simulink model "SF107A_MotRplCoggCmd"  (R2013b)
settings: Solver=FixedStepDiscrete  SolverMode=SingleTasking  StartTime=0.0  StopTime=1  FixedStep=0.002  RelTol=1e-3
values from neighbouring files (symbols this model uses):
  ARCHGLBPRM_2PI_ULS_F32 = DataDict.Constant    [SF107A_MotRplCoggCmd_DataDict.m]
  ARCHGLBPRM_FLOATZEROTHD_ULS_F32 = DataDict.Constant    [SF107A_MotRplCoggCmd_DataDict.m]
  ININITRNIDXCON_CNT_U16 = DataDict.Constant    [SF107A_MotRplCoggCmd_DataDict.m]
  ITRNIDXCON_CNT_U08 = DataDict.Constant    [SF107A_MotRplCoggCmd_DataDict.m]
  MotRplCoggCmdHrmncOrder1Elec = DataDict.Calibration    [SF107A_MotRplCoggCmd_DataDict.m]
  MotRplCoggCmdHrmncOrder2Elec = DataDict.Calibration    [SF107A_MotRplCoggCmd_DataDict.m]
  MotRplCoggCmdHrmncOrder3Elec = DataDict.Calibration    [SF107A_MotRplCoggCmd_DataDict.m]
  ONEOVER12_MOTREV_F32 = DataDict.Constant    [SF107A_MotRplCoggCmd_DataDict.m]
  ONEOVER2_ULS_F32 = DataDict.Constant    [SF107A_MotRplCoggCmd_DataDict.m]
  ONEOVER2PI_ULS_F32 = DataDict.Constant    [SF107A_MotRplCoggCmd_DataDict.m]
  ONEOVER4_ULS_F32 = DataDict.Constant    [SF107A_MotRplCoggCmd_DataDict.m]
  SINCNVNCON1_ULS_F32 = DataDict.Constant    [SF107A_MotRplCoggCmd_DataDict.m]
  SINCNVNCON2_ULS_F32 = DataDict.Constant    [SF107A_MotRplCoggCmd_DataDict.m]
  SINCNVNCONTBL_ULS_U16 = DataDict.Constant    [SF107A_MotRplCoggCmd_DataDict.m]
undefined symbols (not defined in the file or in its folder): NvmGetErrSts1
libraries: FloatToFixd x8, FixdToFloat x8, NxtrNvM x3, NxtrLim x3, simulink x2, NxtrAbslt x1
(part 1 of 3)
settings Model: Creator=BZHF94  LastModifiedBy=BZHF94
settings SolverCC: AutoInsertRateTranBlk=on  InsertRTBMode=Always
settings DataIOCC: LimitDataPoints=off  SaveFormat=Structure  ReturnWorkspaceOutputs=on
settings OptimizationCC: BlockReduction=off  InlineParams=on  ZeroExternalMemoryAtStartup=off  ZeroInternalMemoryAtStartup=off  OptimizeModelRefInitCode=on  LifeSpan=1
settings DebuggingCC: SignalInfNanChecking=error  SignalRangeChecking=warning  UnderspecifiedInitializationDetection=Simplified  SolverPrmCheckMsg=error  InheritedTsInSrcMsg=error  DiscreteInheritContinuousMsg=error  SingleTaskRateTransMsg=error  TasksWithSamePriorityMsg=error  SigSpecEnsureSampleTimeMsg=error  CheckMatrixSingularityMsg=error  ParameterUnderflowMsg=error  ParameterPrecisionLossMsg=error  ParameterTunabilityLossMsg=error  FixptConstUnderflowMsg=warning  FixptConstOverflowMsg=warning  VectorMatrixConversionMsg=error  SignalLabelMismatchMsg=error  UnconnectedInputMsg=error  UnconnectedOutputMsg=error  UnconnectedLineMsg=error  SFcnCompatibilityMsg=error  UniqueDataStoreMsg=warning  BusObjectLabelMismatch=error  RootOutportRequireBusObject=error  AssertControl=DisableAll  ModelReferenceIOMsg=error  ModelReferenceVersionMismatchMessage=warning  ModelReferenceIOMismatchMessage=error  ModelReferenceCSMismatchMessage=warning  ModelReferenceDataLoggingMessage=error  StateNameClashWarn=warning  StrictBusMsg=ErrorOnBusTreatedAsVector  NonBusSignalsTreatedAsBus=error  SFUnexpectedBacktrackingDiag=error  SFInvalidInputDataAccessInChartInitDiag=error  SFNoUnconditionalDefaultTransitionDiag=error  SFTransitionOutsideNaturalParentDiag=error  SFUnconditionalTransitionShadowingDiag=error  SFUndirectedBroadcastEventsDiag=error
settings ModelReferenceCC: ModelReferenceNumInstancesAllowed=Single
settings RTWCC: SystemTargetFile=autosar.tlc  GenCodeOnly=on  TemplateMakefile=ert_default_tmf  Description=AUTOSAR  GenerateReport=on  ProcessScript=autosar_make_rtw_hook  LaunchReport=on
settings CodeAppCC: GenerateComments=off  IgnoreCustomStorageClasses=off  CustomSymbolStrType=$N$R$M  CustomSymbolStrBlkIO=$N$M  SimulinkBlockComments=off
settings STFCustomTargetCC: ParMdlRefBuildCompliant=on  CompOptLevelCompliant=on  IncludeMdlTerminateFcn=off  CombineOutputUpdateFcns=on  SuppressErrorStatus=on  ERTFirstTimeCompliant=on  ERTCustomFileBanners=on  SupportNonFinite=off  SupportComplex=off  SupportContinuousTime=off  SupportNonInlinedSFcns=off  MATLABClassNameForMDSCustomization=Simulink.SoftwareTarget.ERTCustomization  AutosarCompliant=on  GRTInterface=off  SystemTargetFile=autosar.tlc
settings ERTTargetCC: CodeReplacementLibrary=ANSI_C  ConcurrentExecutionCompliant=off  IncludeMdlTerminateFcn=off  SuppressErrorStatus=on  SupportNonFinite=off  SupportComplex=off  ModelStepFunctionPrototypeControlCompliant=off  CPPClassGenCompliant=off  AutosarCompliant=on  InlinedParameterPlacement=NonHierarchical  ERTCustomFileTemplate=example_file_process.tlc  EnableUserReplacementTypes=on

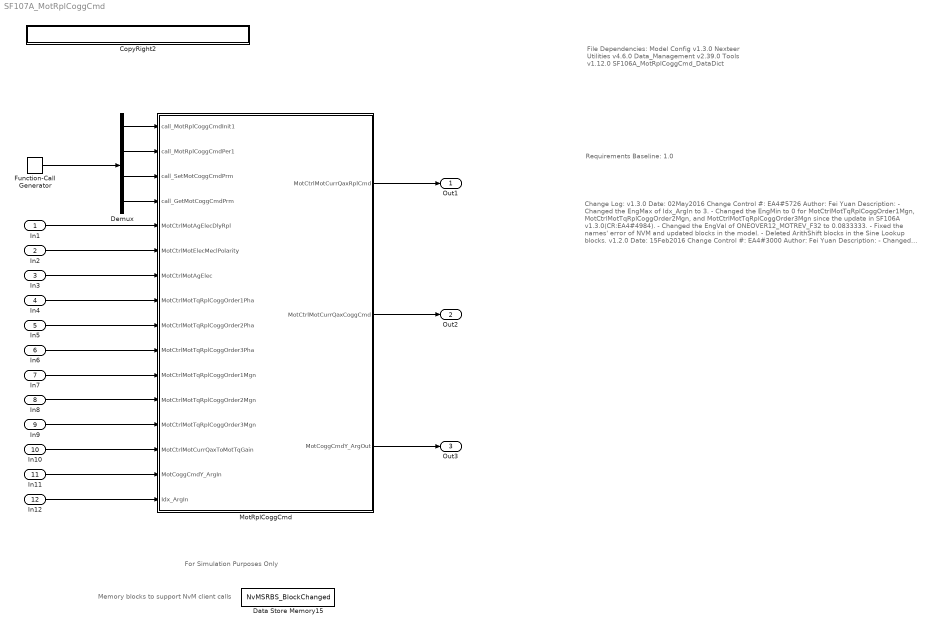
== system SF107A_MotRplCoggCmd ==
  note: Change Log:
      |
      | v1.3.0
      | Date: 02May2016
      | Change Control #: EA4#5726
      | Author: Fei Yuan
      | Description:
      | - Changed the EngMax of Idx_ArgIn to 3.
      | - Changed the EngMin to 0 for MotCtrlMotTqRplCoggOrder1Mgn,
      |   MotCtrlMotTqRplCoggOrder2Mgn, and MotCtrlMotTqRplCoggOrder3Mgn
      |   since the update in SF106A v1.3.0(CR:EA4#4984).
      | - Changed the EngVal of ONEOVER12_MOTREV_F32 to 0.0833333.
      | - Fixed the names' error of NVM and updated blocks in the model.
      | - Deleted ArithShift blocks in the Sine Lookup blocks.
      |
      |
      | v1.2.0
      | Date: 15Feb2016
      | Change Control #: EA4#3000
      | Author: Fei Yuan
      | Description:
      | - Changed the logic of wrapping block to fix the floating point exception.
      |
      |
      | v1.1.0
      | Date: 11February2016
      | Change Control #: EA4#3000
      | Author: Fei Yuan
      | Description:
      | - Change Per1 context to "Non-Rte".
      | - Add "MotRplCoggCmdInit1" to SetRamBlockStatus CallLocation
      | - Correct the MOTRPLCMDHILIM_AMPR_F32.EngMax to 29.
      | - Delete COGGIDXCON_CNT_U16 and MOTCOGGCMDY_MOTNWTMTR_S1P14
      | - Add the Constant ININITRNIDXCON_CNT_U16.
      | - Change the size of SINCNVNCONTBL_ULS_U16 to 513.
      | - Add a missed unary block.
      | - Add new logic in "Convert to 0 to Pi/2" block.
      |
      |
      | v1.0.0
      | Date: 01February2016
      | Change Control #: EA4#3000
      | Author: Fei Yuan
      | Description:
      | - Initial release for EA4 based on version 1 in EA3.
  note: File Dependencies:
      |
      | Model Config v1.3.0
      | Nexteer Utilities v4.6.0
      | Data_Management v2.39.0
      | Tools v1.12.0
      | SF106A_MotRplCoggCmd_DataDict
  note: Requirements Baseline: 1.0
  note: For Simulation Purposes Only
  note: Memory blocks to support NvM client calls
  In1 : Inport
  In2 : Inport  Port=2
  In3 : Inport  Port=3
  In4 : Inport  Port=4
  In5 : Inport  Port=5
  In6 : Inport  Port=6
  In7 : Inport  Port=7
  In8 : Inport  Port=8
  In9 : Inport  Port=9
  In10 : Inport  Port=10
  In11 : Inport  Port=11  OutDataTypeStr=int16
  In12 : Inport  Port=12
  CopyRight2 : Subsystem  Description=|  mask(Copyright Information){none=on}
      | Copyright info block.                                               
      |                                                                     
      | Place copyright information at the top of every subsystem in design.
      mask prompts: none "No parameters"
      mask help: Place copyright information at the top of every subsystem in design.
      mask Display:
      | NxtrConf = 'Nexteer Confidential';
      | 
      | sys = bdroot; %handle for the current model ("system")
      | first = get_param(sys,'Created');
      | if(isempty(first))
      |     first = datestr(now,'yyyy');
      | else
      |     first = first(end-3:end);  %year is last four digits
      | end
      | 
      | last = get_param(sys,'LastModifiedDate');
      | if isempty(last)
      |     last = datestr(now,'yyyy');
      | else
      |     last = last(end-3:end);
      | end
      | 
      | if strcmp(first,last)
      |     fprintf('%s -- Copyright %s Nexteer',NxtrConf,first)
      | else
      |     fprintf('%s -- %s%s- %s Nexteer',NxtrConf,char(169),first,last)
      | end
  Data Store Memory15 : DataStoreMemory  DataStoreName=NvMSRBS_BlockChanged  VectorParams1D=off
  Demux : Demux
  Function-Call Generator : simulink/Ports & Subsystems/Function-Call Generator  RequirementInfo={} %GIDa_6477a55e_09d1_416c_bd2a_f96e072289e0  sample_time=1  numberOfIterations=1
  MotRplCoggCmd : Subsystem
  Out1 : Outport
  Out2 : Outport  Port=2
  Out3 : Outport  Port=3
  wires:
  In1/1 -> MotRplCoggCmd/5(MotCtrlMotAgElecDlyRpl)
  In2/1 -> MotRplCoggCmd/6(MotCtrlMotElecMeclPolarity)
  In3/1 -> MotRplCoggCmd/7(MotCtrlMotAgElec)
  In4/1 -> MotRplCoggCmd/8(MotCtrlMotTqRplCoggOrder1Pha)
  In5/1 -> MotRplCoggCmd/9(MotCtrlMotTqRplCoggOrder2Pha)
  In6/1 -> MotRplCoggCmd/10(MotCtrlMotTqRplCoggOrder3Pha)
  In7/1 -> MotRplCoggCmd/11(MotCtrlMotTqRplCoggOrder1Mgn)
  In8/1 -> MotRplCoggCmd/12(MotCtrlMotTqRplCoggOrder2Mgn)
  In9/1 -> MotRplCoggCmd/13(MotCtrlMotTqRplCoggOrder3Mgn)
  In10/1 -> MotRplCoggCmd/14(MotCtrlMotCurrQaxToMotTqGain)
  MotRplCoggCmd/1(MotCtrlMotCurrQaxRplCmd) -> Out1/1
  MotRplCoggCmd/2(MotCtrlMotCurrQaxCoggCmd) -> Out2/1
  Function-Call Generator/1 -> Demux/1
  In11/1 -> MotRplCoggCmd/15(MotCoggCmdY_ArgIn)
  In12/1 -> MotRplCoggCmd/16(Idx_ArgIn)
  Demux/3 -> MotRplCoggCmd/3(call_SetMotCoggCmdPrm)
  Demux/4 -> MotRplCoggCmd/4(call_GetMotCoggCmdPrm)
  Demux/2 -> MotRplCoggCmd/2(call_MotRplCoggCmdPer1)
  Demux/1 -> MotRplCoggCmd/1(call_MotRplCoggCmdInit1)
  MotRplCoggCmd/3(MotCoggCmdY_ArgOut) -> Out3/1

== system SF107A_MotRplCoggCmd/CopyRight2 ==

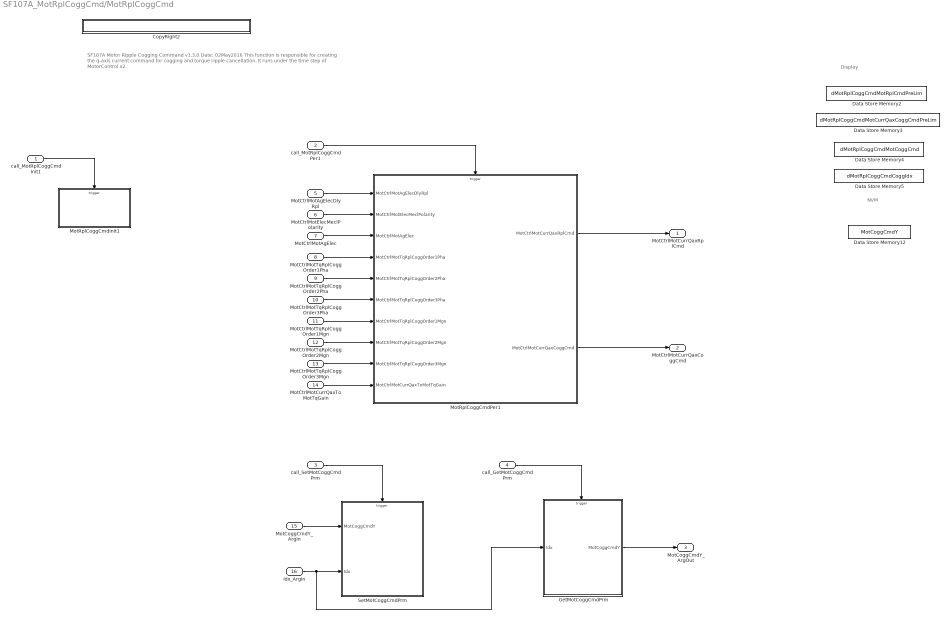
== system SF107A_MotRplCoggCmd/MotRplCoggCmd ==
  note: SF107A  Motor Ripple Cogging Command
      | v1.3.0      Date: 02May2016
      |
      | This function is responsible for creating the q-axis current command for cogging and torque ripple cancellation.
      | It runs under the time step of MotorControl x2.
  note: NVM
  note: Display
  call_MotRplCoggCmdInit1 : Inport
  call_MotRplCoggCmdPer1 : Inport  RequirementInfo="{'linktype_rmi_doors' '0000bb46 (/E-STEER Core/SubSystem Specifications/Application Functions/SF99/SF107A Cogging and Ripple Command Generation)' '#SF107A_49' 'true' 'REQ:  SF107A_49' '' } %GIDa_bcde757e_fcf1_400f_9a5c_d951bd685b53"  Port=2
  call_SetMotCoggCmdPrm : Inport  Port=3
  call_GetMotCoggCmdPrm : Inport  Port=4
  MotCtrlMotAgElecDlyRpl : Inport  RequirementInfo="{'linktype_rmi_doors' '0000bb46 (/E-STEER Core/SubSystem Specifications/Application Functions/SF99/SF107A Cogging and Ripple Command Generation)' '#SF107A_45' 'true' 'REQ:  SF107A_45' '' } %GIDa_759bd4cf_ee1e_4f48_ad2a_68232b25c211"  Port=5
  MotCtrlMotElecMeclPolarity : Inport  RequirementInfo="{'linktype_rmi_doors' '0000bb46 (/E-STEER Core/SubSystem Specifications/Application Functions/SF99/SF107A Cogging and Ripple Command Generation)' '#SF107A_46' 'true' 'REQ:  SF107A_46' '' } %GIDa_d359bdf1_f0a3_4952_a26e_4e6f5812eb7c"  Port=6
  MotCtrlMotAgElec : Inport  RequirementInfo="{'linktype_rmi_doors' '0000bb46 (/E-STEER Core/SubSystem Specifications/Application Functions/SF99/SF107A Cogging and Ripple Command Generation)' '#SF107A_43' 'true' 'REQ:  SF107A_43' '' } %GIDa_21806179_a7db_45e0_974d_baa248ff84af"  Port=7
  MotCtrlMotTqRplCoggOrder1Pha : Inport  RequirementInfo="{'linktype_rmi_doors' '0000bb46 (/E-STEER Core/SubSystem Specifications/Application Functions/SF99/SF107A Cogging and Ripple Command Generation)' '#SF107A_38' 'true' 'REQ:  SF107A_38' '' } %GIDa_76ec82d2_a38c_47ae_b701_241d2d548300"  Port=8
  MotCtrlMotTqRplCoggOrder2Pha : Inport  RequirementInfo="{'linktype_rmi_doors' '0000bb46 (/E-STEER Core/SubSystem Specifications/Application Functions/SF99/SF107A Cogging and Ripple Command Generation)' '#SF107A_40' 'true' 'REQ:  SF107A_40' '' } %GIDa_59edcd68_ad99_42db_8c02_5e556eb509ac"  Port=9
  MotCtrlMotTqRplCoggOrder3Pha : Inport  RequirementInfo="{'linktype_rmi_doors' '0000bb46 (/E-STEER Core/SubSystem Specifications/Application Functions/SF99/SF107A Cogging and Ripple Command Generation)' '#SF107A_42' 'true' 'REQ:  SF107A_42' '' } %GIDa_4883dac2_53a7_4d05_a76a_d63a8a01ae4d"  Port=10
  MotCtrlMotTqRplCoggOrder1Mgn : Inport  RequirementInfo="{'linktype_rmi_doors' '0000bb46 (/E-STEER Core/SubSystem Specifications/Application Functions/SF99/SF107A Cogging and Ripple Command Generation)' '#SF107A_27' 'true' 'REQ:  SF107A_27' '' } %GIDa_75ad0a99_38bc_44be_af39_747cf86f05ec"  Port=11
  MotCtrlMotTqRplCoggOrder2Mgn : Inport  RequirementInfo="{'linktype_rmi_doors' '0000bb46 (/E-STEER Core/SubSystem Specifications/Application Functions/SF99/SF107A Cogging and Ripple Command Generation)' '#SF107A_39' 'true' 'REQ:  SF107A_39' '' } %GIDa_040945aa_cac7_4d8d_86dc_7274d12a7576"  Port=12
  MotCtrlMotTqRplCoggOrder3Mgn : Inport  RequirementInfo="{'linktype_rmi_doors' '0000bb46 (/E-STEER Core/SubSystem Specifications/Application Functions/SF99/SF107A Cogging and Ripple Command Generation)' '#SF107A_41' 'true' 'REQ:  SF107A_41' '' } %GIDa_1dbb5808_0eab_4535_8b60_cc6f49189c56"  Port=13
  MotCtrlMotCurrQaxToMotTqGain : Inport  RequirementInfo="{'linktype_rmi_doors' '0000bb46 (/E-STEER Core/SubSystem Specifications/Application Functions/SF99/SF107A Cogging and Ripple Command Generation)' '#SF107A_44' 'true' 'REQ:  SF107A_44' '' } %GIDa_8093fd36_868b_4102_b9e2_e2b5f3d0e07d"  Port=14
  MotCoggCmdY_ArgIn : Inport  Port=15
  Idx_ArgIn : Inport  Port=16
  CopyRight2 : Subsystem  Description=|  mask(Copyright Information){none=on}
      | Copyright info block.                                               
      |                                                                     
      | Place copyright information at the top of every subsystem in design.
      mask prompts: none "No parameters"
      mask help: Place copyright information at the top of every subsystem in design.
      mask Display:
      | NxtrConf = 'Nexteer Confidential';
      | 
      | sys = bdroot; %handle for the current model ("system")
      | first = get_param(sys,'Created');
      | if(isempty(first))
      |     first = datestr(now,'yyyy');
      | else
      |     first = first(end-3:end);  %year is last four digits
      | end
      | 
      | last = get_param(sys,'LastModifiedDate');
      | if isempty(last)
      |     last = datestr(now,'yyyy');
      | else
      |     last = last(end-3:end);
      | end
      | 
      | if strcmp(first,last)
      |     fprintf('%s -- Copyright %s Nexteer',NxtrConf,first)
      | else
      |     fprintf('%s -- %s%s- %s Nexteer',NxtrConf,char(169),first,last)
      | end
  Data Store Memory12 : DataStoreMemory  DataStoreName=MotCoggCmdY  InitialValue=[]  OutDataTypeStr=int16  StateMustResolveToSignalObject=on
  Data Store Memory2 : DataStoreMemory  DataStoreName=dMotRplCoggCmdMotRplCmdPreLim  InitialValue=[]  VectorParams1D=off  StateMustResolveToSignalObject=on
  Data Store Memory3 : DataStoreMemory  DataStoreName=dMotRplCoggCmdMotCurrQaxCoggCmdPreLim  InitialValue=[]  VectorParams1D=off  StateMustResolveToSignalObject=on
  Data Store Memory4 : DataStoreMemory  DataStoreName=dMotRplCoggCmdMotCoggCmd  InitialValue=[]  VectorParams1D=off  StateMustResolveToSignalObject=on
  Data Store Memory5 : DataStoreMemory  DataStoreName=dMotRplCoggCmdCoggIdx  InitialValue=[]  VectorParams1D=off  StateMustResolveToSignalObject=on
  GetMotCoggCmdPrm : Subsystem
  MotRplCoggCmdInit1 : Subsystem
  MotRplCoggCmdPer1 : Subsystem
  SetMotCoggCmdPrm : Subsystem
  MotCtrlMotCurrQaxRplCmd : Outport  RequirementInfo="{'linktype_rmi_doors' '0000bb46 (/E-STEER Core/SubSystem Specifications/Application Functions/SF99/SF107A Cogging and Ripple Command Generation)' '#SF107A_47' 'true' 'REQ:  SF107A_47' '' } %GIDa_c223fd26_86db_4771_9987_8f6635ad3f76"
  MotCtrlMotCurrQaxCoggCmd : Outport  RequirementInfo="{'linktype_rmi_doors' '0000bb46 (/E-STEER Core/SubSystem Specifications/Application Functions/SF99/SF107A Cogging and Ripple Command Generation)' '#SF107A_28' 'true' 'REQ:  SF107A_28' '' } %GIDa_efe72f72_a005_42fa_9193_c14ee39dea59"  Port=2
  MotCoggCmdY_ArgOut : Outport  Port=3
  wires:
  MotCtrlMotAgElecDlyRpl/1 -> MotRplCoggCmdPer1/1(MotCtrlMotAgElecDlyRpl)
  MotCtrlMotElecMeclPolarity/1 -> MotRplCoggCmdPer1/2(MotCtrlMotElecMeclPolarity)
  MotCtrlMotAgElec/1 -> MotRplCoggCmdPer1/3(MotCtrlMotAgElec)
  MotCtrlMotTqRplCoggOrder1Pha/1 -> MotRplCoggCmdPer1/4(MotCtrlMotTqRplCoggOrder1Pha)
  MotCtrlMotTqRplCoggOrder2Pha/1 -> MotRplCoggCmdPer1/5(MotCtrlMotTqRplCoggOrder2Pha)
  MotCtrlMotTqRplCoggOrder3Pha/1 -> MotRplCoggCmdPer1/6(MotCtrlMotTqRplCoggOrder3Pha)
  MotCtrlMotTqRplCoggOrder1Mgn/1 -> MotRplCoggCmdPer1/7(MotCtrlMotTqRplCoggOrder1Mgn)
  MotCtrlMotTqRplCoggOrder2Mgn/1 -> MotRplCoggCmdPer1/8(MotCtrlMotTqRplCoggOrder2Mgn)
  MotCtrlMotTqRplCoggOrder3Mgn/1 -> MotRplCoggCmdPer1/9(MotCtrlMotTqRplCoggOrder3Mgn)
  MotCtrlMotCurrQaxToMotTqGain/1 -> MotRplCoggCmdPer1/10(MotCtrlMotCurrQaxToMotTqGain)
  MotRplCoggCmdPer1/1(MotCtrlMotCurrQaxRplCmd) -> MotCtrlMotCurrQaxRplCmd/1
  MotRplCoggCmdPer1/2(MotCtrlMotCurrQaxCoggCmd) -> MotCtrlMotCurrQaxCoggCmd/1
  call_MotRplCoggCmdPer1/1 -> MotRplCoggCmdPer1/Trigger
  call_MotRplCoggCmdInit1/1 -> MotRplCoggCmdInit1/Trigger
  call_SetMotCoggCmdPrm/1 -> SetMotCoggCmdPrm/Trigger
  call_GetMotCoggCmdPrm/1 -> GetMotCoggCmdPrm/Trigger
  Idx_ArgIn/1 -> GetMotCoggCmdPrm/1(Idx), SetMotCoggCmdPrm/2(Idx)
  MotCoggCmdY_ArgIn/1 -> SetMotCoggCmdPrm/1(MotCoggCmdY)
  GetMotCoggCmdPrm/1(MotCoggCmdY) -> MotCoggCmdY_ArgOut/1

== system SF107A_MotRplCoggCmd/MotRplCoggCmd/CopyRight2 ==

== system SF107A_MotRplCoggCmd/MotRplCoggCmd/GetMotCoggCmdPrm ==
  Idx : Inport
  function : TriggerPort  TriggerType=function-call
  Constant1 : Constant  Value=ITRNIDXCON_CNT_U08  OutDataTypeStr=int16
  CopyRight1 : Subsystem  Description=|  mask(Copyright Information){none=on}
      | Copyright info block.                                               
      |                                                                     
      | Place copyright information at the top of every subsystem in design.
      mask prompts: none "No parameters"
      mask help: Place copyright information at the top of every subsystem in design.
      mask Display:
      | NxtrConf = 'Nexteer Confidential';
      | 
      | sys = bdroot; %handle for the current model ("system")
      | first = get_param(sys,'Created');
      | if(isempty(first))
      |     first = datestr(now,'yyyy');
      | else
      |     first = first(end-3:end);  %year is last four digits
      | end
      | 
      | last = get_param(sys,'LastModifiedDate');
      | if isempty(last)
      |     last = datestr(now,'yyyy');
      | else
      |     last = last(end-3:end);
      | end
      | 
      | if strcmp(first,last)
      |     fprintf('%s -- Copyright %s Nexteer',NxtrConf,first)
      | else
      |     fprintf('%s -- %s%s- %s Nexteer',NxtrConf,char(169),first,last)
      | end
  For Iterator Subsystem : Subsystem  RequirementInfo="{'linktype_rmi_doors' '0000bb46 (/E-STEER Core/SubSystem Specifications/Application Functions/SF99/SF107A Cogging and Ripple Command Generation)' '#SF107A_33' 'true' 'REQ:  SF107A_33' '' } %GIDa_45473554_817e_49b7_8dca_101340bc12f0"  TreatAsAtomicUnit=on
  MotCoggCmdY : Outport
  wires:
  Idx/1 -> For Iterator Subsystem/1(Idx)
  For Iterator Subsystem/1(MotCoggCmdY) -> MotCoggCmdY/1
  Constant1/1 -> For Iterator Subsystem/2(ItrnIdxCon)

== system SF107A_MotRplCoggCmd/MotRplCoggCmd/MotRplCoggCmdInit1 ==
  function : TriggerPort  TriggerType=function-call
  CopyRight2 : Subsystem  Description=|  mask(Copyright Information){none=on}
      | Copyright info block.                                               
      |                                                                     
      | Place copyright information at the top of every subsystem in design.
      mask prompts: none "No parameters"
      mask help: Place copyright information at the top of every subsystem in design.
      mask Display:
      | NxtrConf = 'Nexteer Confidential';
      | 
      | sys = bdroot; %handle for the current model ("system")
      | first = get_param(sys,'Created');
      | if(isempty(first))
      |     first = datestr(now,'yyyy');
      | else
      |     first = first(end-3:end);  %year is last four digits
      | end
      | 
      | last = get_param(sys,'LastModifiedDate');
      | if isempty(last)
      |     last = datestr(now,'yyyy');
      | else
      |     last = last(end-3:end);
      | end
      | 
      | if strcmp(first,last)
      |     fprintf('%s -- Copyright %s Nexteer',NxtrConf,first)
      | else
      |     fprintf('%s -- %s%s- %s Nexteer',NxtrConf,char(169),first,last)
      | end
  Data Type Conversion : DataTypeConversion  RequirementInfo="{'linktype_rmi_doors' '0000bb46 (/E-STEER Core/SubSystem Specifications/Application Functions/SF99/SF107A Cogging and Ripple Command Generation)' '#SF107A_61' 'true' 'REQ:  SF107A_61' '' } %GIDa_7543bd06_1602_4119_b52d_e662400f79a4"  OutDataTypeStr=int32
  Data Type Conversion1 : DataTypeConversion  RequirementInfo="{'linktype_rmi_doors' '0000bb46 (/E-STEER Core/SubSystem Specifications/Application Functions/SF99/SF107A Cogging and Ripple Command Generation)' '#SF107A_61' 'true' 'REQ:  SF107A_61' '' } %GIDa_e4f111be_1c13_4101_a6fe_36d4dd11c4c4"  OutDataTypeStr=Enum: NvmGetErrSts1
  Enumerated Constant : simulink/Sources/Enumerated Constant  RequirementInfo="{'linktype_rmi_doors' '0000bb46 (/E-STEER Core/SubSystem Specifications/Application Functions/SF99/SF107A Cogging and Ripple Command Generation)' '#SF107A_61' 'true' 'REQ:  SF107A_61' '' } %GIDa_6ad17a04_5c1e_4dc7_8ab4_71a48d0dc388"  OutDataTypeStr=Enum: NvmGetErrSts1  Value=NvmGetErrSts1.REQUEST_OK  SampleTime=inf
  Get Error Status : NxtrNvM/Get Error Status  RequirementInfo="{'linktype_rmi_doors' '0000bb46 (/E-STEER Core/SubSystem Specifications/Application Functions/SF99/SF107A Cogging and Ripple Command Generation)' '#SF107A_61' 'true' 'REQ:  SF107A_61' '' } %GIDa_e572d21d_63bd_432d_baf2_5c021ad23777"  FuncName=Get Error Status  NvMBlockName=MotCoggCmdY  VoidFuncRtn=on  ReqResPtr_DSN=NvMGES_ReqResPtr  Return_DSN=NvMGES_ReqResPtr
      settings: AttributesFormatString=%<FuncName>
  If : If  RequirementInfo="{'linktype_rmi_doors' '0000bb46 (/E-STEER Core/SubSystem Specifications/Application Functions/SF99/SF107A Cogging and Ripple Command Generation)' '#SF107A_61' 'true' 'REQ:  SF107A_61' '' } %GIDa_e4fe0c89_1c6e_4333_af03_6094cd431682"  IfExpression=u1  ShowElse=off
  NVM is NOT okay : Subsystem  RequirementInfo="{'linktype_rmi_doors' '0000bb46 (/E-STEER Core/SubSystem Specifications/Application Functions/SF99/SF107A Cogging and Ripple Command Generation)' '#SF107A_61' 'true' 'REQ:  SF107A_61' '' } %GIDa_2b24311b_dea0_4c39_b838_f46fba703cea"  TreatAsAtomicUnit=on
  Relational Operator : RelationalOperator  RequirementInfo="{'linktype_rmi_doors' '0000bb46 (/E-STEER Core/SubSystem Specifications/Application Functions/SF99/SF107A Cogging and Ripple Command Generation)' '#SF107A_61' 'true' 'REQ:  SF107A_61' '' } %GIDa_be3389a3_2489_4935_b3c7_7ac566e8e832"  Operator=~=  OutDataTypeStr=boolean
  wires:
  Get Error Status/1 -> Data Type Conversion/1
  If/1 -> NVM is NOT okay/Action
  Enumerated Constant/1 -> Relational Operator/2
  Relational Operator/1 -> If/1
  Data Type Conversion/1 -> Data Type Conversion1/1
  Data Type Conversion1/1 -> Relational Operator/1

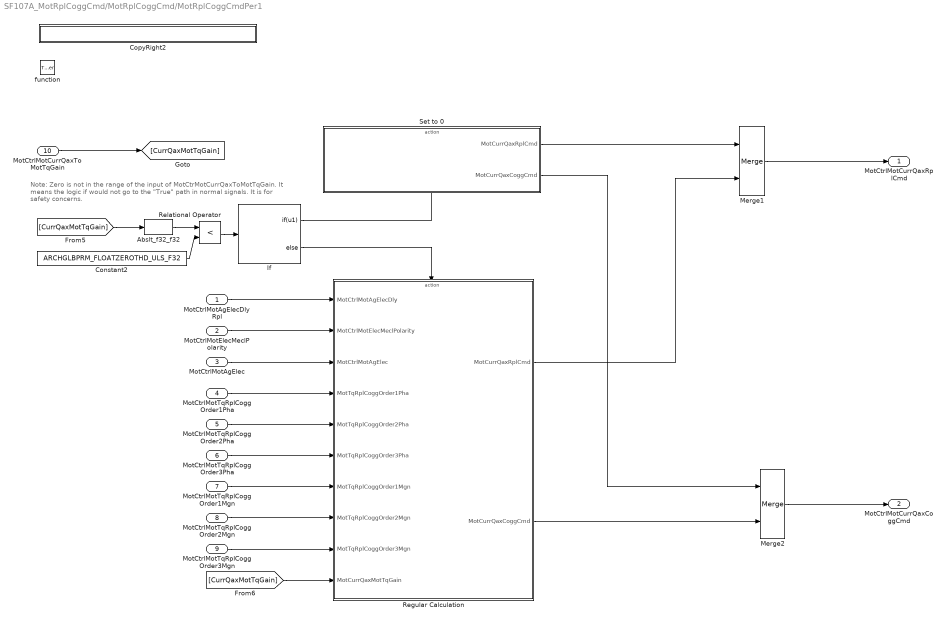
== system SF107A_MotRplCoggCmd/MotRplCoggCmd/MotRplCoggCmdPer1 ==
  note: Note: Zero is not in the range of the input of MotCtrMotCurrQaxToMotTqGain.
      | It means the logic if would not go to the "True" path in normal signals. It is for
      | safety concerns.
  MotCtrlMotAgElecDlyRpl : Inport
  MotCtrlMotElecMeclPolarity : Inport  Port=2
  MotCtrlMotAgElec : Inport  Port=3
  MotCtrlMotTqRplCoggOrder1Pha : Inport  Port=4
  MotCtrlMotTqRplCoggOrder2Pha : Inport  Port=5
  MotCtrlMotTqRplCoggOrder3Pha : Inport  Port=6
  MotCtrlMotTqRplCoggOrder1Mgn : Inport  Port=7
  MotCtrlMotTqRplCoggOrder2Mgn : Inport  Port=8
  MotCtrlMotTqRplCoggOrder3Mgn : Inport  Port=9
  MotCtrlMotCurrQaxToMotTqGain : Inport  Port=10
  function : TriggerPort  TriggerType=function-call
  Abslt_f32_f32 : NxtrAbslt/Abslt_f32_f32  RequirementInfo="{'linktype_rmi_doors' '0000bb46 (/E-STEER Core/SubSystem Specifications/Application Functions/SF99/SF107A Cogging and Ripple Command Generation)' '#SF107A_61' 'true' 'REQ:  SF107A_61' '' } %GIDa_98ab6231_9957_4905_8685_e5740981592e"  SFunctionSpec=single y1 = Abslt_f32_f32(single u1)
      settings: AttributesFormatString=%<Name>
  Constant2 : Constant  RequirementInfo="{'linktype_rmi_doors' '0000bb46 (/E-STEER Core/SubSystem Specifications/Application Functions/SF99/SF107A Cogging and Ripple Command Generation)' '#SF107A_61' 'true' 'REQ:  SF107A_61' '' } %GIDa_2b46aefd_770c_4243_8404_9e28f4c01df7"  Value=ARCHGLBPRM_FLOATZEROTHD_ULS_F32
  CopyRight2 : Subsystem  Description=|  mask(Copyright Information){none=on}
      | Copyright info block.                                               
      |                                                                     
      | Place copyright information at the top of every subsystem in design.
      mask prompts: none "No parameters"
      mask help: Place copyright information at the top of every subsystem in design.
      mask Display:
      | NxtrConf = 'Nexteer Confidential';
      | 
      | sys = bdroot; %handle for the current model ("system")
      | first = get_param(sys,'Created');
      | if(isempty(first))
      |     first = datestr(now,'yyyy');
      | else
      |     first = first(end-3:end);  %year is last four digits
      | end
      | 
      | last = get_param(sys,'LastModifiedDate');
      | if isempty(last)
      |     last = datestr(now,'yyyy');
      | else
      |     last = last(end-3:end);
      | end
      | 
      | if strcmp(first,last)
      |     fprintf('%s -- Copyright %s Nexteer',NxtrConf,first)
      | else
      |     fprintf('%s -- %s%s- %s Nexteer',NxtrConf,char(169),first,last)
      | end
  If : If  RequirementInfo="{'linktype_rmi_doors' '0000bb46 (/E-STEER Core/SubSystem Specifications/Application Functions/SF99/SF107A Cogging and Ripple Command Generation)' '#SF107A_61' 'true' 'REQ:  SF107A_61' '' } %GIDa_3a5860a3_0e2e_4331_aab2_e5b66dff5352"  IfExpression=u1
  Merge1 : Merge  RequirementInfo="{'linktype_rmi_doors' '0000bb46 (/E-STEER Core/SubSystem Specifications/Application Functions/SF99/SF107A Cogging and Ripple Command Generation)' '#SF107A_61' 'true' 'REQ:  SF107A_61' '' } %GIDa_c1020c94_da0e_48f1_812f_751dd1c0e521"
  Merge2 : Merge  RequirementInfo="{'linktype_rmi_doors' '0000bb46 (/E-STEER Core/SubSystem Specifications/Application Functions/SF99/SF107A Cogging and Ripple Command Generation)' '#SF107A_61' 'true' 'REQ:  SF107A_61' '' } %GIDa_d62df4b8_5fb9_4378_80e2_de7400452455"
  Regular Calculation : Subsystem  TreatAsAtomicUnit=on
  Relational Operator : RelationalOperator  RequirementInfo="{'linktype_rmi_doors' '0000bb46 (/E-STEER Core/SubSystem Specifications/Application Functions/SF99/SF107A Cogging and Ripple Command Generation)' '#SF107A_61' 'true' 'REQ:  SF107A_61' '' } %GIDa_0649a214_7cff_4b5d_92b0_ac2271458f93"  Operator=<  OutDataTypeStr=boolean
  Set to 0 : Subsystem  RequirementInfo="{'linktype_rmi_doors' '0000bb46 (/E-STEER Core/SubSystem Specifications/Application Functions/SF99/SF107A Cogging and Ripple Command Generation)' '#SF107A_61' 'true' 'REQ:  SF107A_61' '' } %GIDa_9ff30e71_4fe0_4a1e_8972_6be45b96b5b5"  TreatAsAtomicUnit=on
  MotCtrlMotCurrQaxRplCmd : Outport
  MotCtrlMotCurrQaxCoggCmd : Outport  Port=2
  wires:
  [CurrQaxMotTqGain] -> Abslt_f32_f32/1
  If/1 -> Set to 0/Action
  If/2 -> Regular Calculation/Action
  Merge1/1 -> MotCtrlMotCurrQaxRplCmd/1
  Merge2/1 -> MotCtrlMotCurrQaxCoggCmd/1
  MotCtrlMotAgElecDlyRpl/1 -> Regular Calculation/1(MotCtrlMotAgElecDly)
  MotCtrlMotElecMeclPolarity/1 -> Regular Calculation/2(MotCtrlMotElecMeclPolarity)
  MotCtrlMotAgElec/1 -> Regular Calculation/3(MotCtrlMotAgElec)
  [CurrQaxMotTqGain] -> Regular Calculation/10(MotCurrQaxMotTqGain)
  MotCtrlMotTqRplCoggOrder1Pha/1 -> Regular Calculation/4(MotTqRplCoggOrder1Pha)
  MotCtrlMotTqRplCoggOrder2Pha/1 -> Regular Calculation/5(MotTqRplCoggOrder2Pha)
  MotCtrlMotTqRplCoggOrder2Mgn/1 -> Regular Calculation/8(MotTqRplCoggOrder2Mgn)
  MotCtrlMotTqRplCoggOrder3Mgn/1 -> Regular Calculation/9(MotTqRplCoggOrder3Mgn)
  MotCtrlMotTqRplCoggOrder1Mgn/1 -> Regular Calculation/7(MotTqRplCoggOrder1Mgn)
  MotCtrlMotTqRplCoggOrder3Pha/1 -> Regular Calculation/6(MotTqRplCoggOrder3Pha)
  Set to 0/1(MotCurrQaxRplCmd) -> Merge1/1
  Set to 0/2(MotCurrQaxCoggCmd) -> Merge2/1
  Regular Calculation/1(MotCurrQaxRplCmd) -> Merge1/2
  Regular Calculation/2(MotCurrQaxCoggCmd) -> Merge2/2
  MotCtrlMotCurrQaxToMotTqGain/1 -> [CurrQaxMotTqGain]
  Constant2/1 -> Relational Operator/2
  Relational Operator/1 -> If/1
  Abslt_f32_f32/1 -> Relational Operator/1

== system SF107A_MotRplCoggCmd/MotRplCoggCmd/SetMotCoggCmdPrm ==
  MotCoggCmdY : Inport
  Idx : Inport  Port=2
  function : TriggerPort  TriggerType=function-call
  Constant : Constant  RequirementInfo="{'linktype_rmi_doors' '0000bb46 (/E-STEER Core/SubSystem Specifications/Application Functions/SF99/SF107A Cogging and Ripple Command Generation)' '#SF107A_61' 'true' 'REQ:  SF107A_61' '' } %GIDa_b2ba887a_b6a1_4ade_ae65_3d5e35303afc"  OutDataTypeStr=double
      settings: AttributesFormatString=%<OutDataTypeStr>
  Constant1 : Constant  Value=ITRNIDXCON_CNT_U08  OutDataTypeStr=int16
  CopyRight1 : Subsystem  Description=|  mask(Copyright Information){none=on}
      | Copyright info block.                                               
      |                                                                     
      | Place copyright information at the top of every subsystem in design.
      mask prompts: none "No parameters"
      mask help: Place copyright information at the top of every subsystem in design.
      mask Display:
      | NxtrConf = 'Nexteer Confidential';
      | 
      | sys = bdroot; %handle for the current model ("system")
      | first = get_param(sys,'Created');
      | if(isempty(first))
      |     first = datestr(now,'yyyy');
      | else
      |     first = first(end-3:end);  %year is last four digits
      | end
      | 
      | last = get_param(sys,'LastModifiedDate');
      | if isempty(last)
      |     last = datestr(now,'yyyy');
      | else
      |     last = last(end-3:end);
      | end
      | 
      | if strcmp(first,last)
      |     fprintf('%s -- Copyright %s Nexteer',NxtrConf,first)
      | else
      |     fprintf('%s -- %s%s- %s Nexteer',NxtrConf,char(169),first,last)
      | end
  For Iterator Subsystem1 : Subsystem  RequirementInfo="{'linktype_rmi_doors' '0000bb46 (/E-STEER Core/SubSystem Specifications/Application Functions/SF99/SF107A Cogging and Ripple Command Generation)' '#SF107A_32' 'true' 'REQ:  SF107A_32' '' } %GIDa_428cf9f1_ea1c_4fc8_a84e_dba4a10a7f1f"  TreatAsAtomicUnit=on
  Set Ram Block Status : NxtrNvM/Set Ram Block Status  RequirementInfo="{'linktype_rmi_doors' '0000bb46 (/E-STEER Core/SubSystem Specifications/Application Functions/SF99/SF107A Cogging and Ripple Command Generation)' '#SF107A_61' 'true' 'REQ:  SF107A_61' '' } %GIDa_b8a29836_1b5e_408e_b699_aa38fbb79f42"  FuncName=Set Ram Block Status  NvMBlockName=MotCoggCmdY  VoidFuncRtn=on  BlockChanged_DSN=NvMSRBS_BlockChanged  Return_DSN=NvMSRBS_Return
      settings: AttributesFormatString=%<FuncName>
  wires:
  Idx/1 -> For Iterator Subsystem1/2(Idx)
  Constant/1 -> Set Ram Block Status/1
  MotCoggCmdY/1 -> For Iterator Subsystem1/1(MotCoggCmdY)
  Constant1/1 -> For Iterator Subsystem1/3(ItrnIdxCon)

== system SF107A_MotRplCoggCmd/MotRplCoggCmd/GetMotCoggCmdPrm/CopyRight1 ==

== system SF107A_MotRplCoggCmd/MotRplCoggCmd/GetMotCoggCmdPrm/For Iterator Subsystem ==
  Idx : Inport
  ItrnIdxCon : Inport  Port=2
  Add : Sum
  Assignment : Assignment  IndexMode=Zero-based  OutputInitialize=Specify size for each dimension in table  IndexOptions=Index vector (port)  Indices=1  OutputSizes=128
  CopyRight1 : Subsystem  Description=|  mask(Copyright Information){none=on}
      | Copyright info block.                                               
      |                                                                     
      | Place copyright information at the top of every subsystem in design.
      mask prompts: none "No parameters"
      mask help: Place copyright information at the top of every subsystem in design.
      mask Display:
      | NxtrConf = 'Nexteer Confidential';
      | 
      | sys = bdroot; %handle for the current model ("system")
      | first = get_param(sys,'Created');
      | if(isempty(first))
      |     first = datestr(now,'yyyy');
      | else
      |     first = first(end-3:end);  %year is last four digits
      | end
      | 
      | last = get_param(sys,'LastModifiedDate');
      | if isempty(last)
      |     last = datestr(now,'yyyy');
      | else
      |     last = last(end-3:end);
      | end
      | 
      | if strcmp(first,last)
      |     fprintf('%s -- Copyright %s Nexteer',NxtrConf,first)
      | else
      |     fprintf('%s -- %s%s- %s Nexteer',NxtrConf,char(169),first,last)
      | end
  Data Store Read2 : DataStoreRead  DataStoreName=MotCoggCmdY
  For Iterator : ForIterator  IterationSource=external  IterationLimit=127  IndexMode=Zero-based  IterationVariableDataType=int16
  Product : Product
  Selector : Selector  IndexMode=Zero-based  InputPortWidth=512  IndexOptions=Index vector (port)  Indices=[1 3]  OutputSizes=1
  MotCoggCmdY : Outport
  wires:
  Selector/1 -> Assignment/1
  Add/1 -> Selector/2
  Idx/1 -> Product/1
  ItrnIdxCon/1 -> Product/2, For Iterator/1
  Product/1 -> Add/1
  For Iterator/1 -> Assignment/2, Add/2
  Assignment/1 -> MotCoggCmdY/1
  Data Store Read2/1 -> Selector/1

== system SF107A_MotRplCoggCmd/MotRplCoggCmd/MotRplCoggCmdInit1/CopyRight2 ==

== system SF107A_MotRplCoggCmd/MotRplCoggCmd/MotRplCoggCmdInit1/NVM is NOT okay ==
  note: NVM is NOT okay. Use calibration values.
  Action Port : ActionPort  ActionType=then
  Constant : Constant  RequirementInfo={} %GIDa_c80d95e7_fa49_477d_b637_4a5240e22e0b
  Constant2 : Constant  RequirementInfo={} %GIDa_4e6b91e3_b9dc_406d_97ac_1e2a3dbe5b79  Value=ININITRNIDXCON_CNT_U16
  CopyRight2 : Subsystem  Description=|  mask(Copyright Information){none=on}
      | Copyright info block.                                               
      |                                                                     
      | Place copyright information at the top of every subsystem in design.
      mask prompts: none "No parameters"
      mask help: Place copyright information at the top of every subsystem in design.
      mask Display:
      | NxtrConf = 'Nexteer Confidential';
      | 
      | sys = bdroot; %handle for the current model ("system")
      | first = get_param(sys,'Created');
      | if(isempty(first))
      |     first = datestr(now,'yyyy');
      | else
      |     first = first(end-3:end);  %year is last four digits
      | end
      | 
      | last = get_param(sys,'LastModifiedDate');
      | if isempty(last)
      |     last = datestr(now,'yyyy');
      | else
      |     last = last(end-3:end);
      | end
      | 
      | if strcmp(first,last)
      |     fprintf('%s -- Copyright %s Nexteer',NxtrConf,first)
      | else
      |     fprintf('%s -- %s%s- %s Nexteer',NxtrConf,char(169),first,last)
      | end
  For Iterator Subsystem : Subsystem  TreatAsAtomicUnit=on
  Set Ram Block Status : NxtrNvM/Set Ram Block Status  RequirementInfo={} %GIDa_1abe2172_f0d6_43f8_901a_e29a2f4c8cab  FuncName=Set Ram Block Status  NvMBlockName=MotCoggCmdY  VoidFuncRtn=on  BlockChanged_DSN=NvMSRBS_BlockChanged  Return_DSN=NvMSRBS_Return
      settings: AttributesFormatString=%<FuncName>
  wires:
  Constant/1 -> Set Ram Block Status/1
  Constant2/1 -> For Iterator Subsystem/1(In1)

== system SF107A_MotRplCoggCmd/MotRplCoggCmd/MotRplCoggCmdPer1/CopyRight2 ==

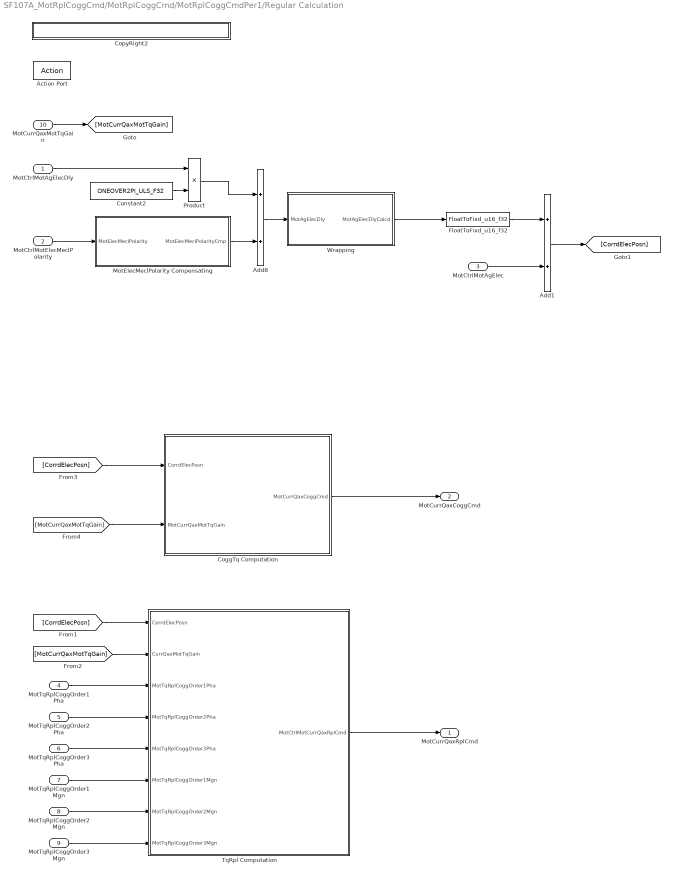
== system SF107A_MotRplCoggCmd/MotRplCoggCmd/MotRplCoggCmdPer1/Regular Calculation ==
  MotCtrlMotAgElecDly : Inport
  MotCtrlMotElecMeclPolarity : Inport  Port=2
  MotCtrlMotAgElec : Inport  RequirementInfo={} %GIDa_c39675f3_ca25_4a4f_a68e_26d18270194e  Port=3
  MotTqRplCoggOrder1Pha : Inport  Port=4
  MotTqRplCoggOrder2Pha : Inport  Port=5
  MotTqRplCoggOrder3Pha : Inport  Port=6
  MotTqRplCoggOrder1Mgn : Inport  Port=7
  MotTqRplCoggOrder2Mgn : Inport  Port=8
  MotTqRplCoggOrder3Mgn : Inport  Port=9
  MotCurrQaxMotTqGain : Inport  Port=10
  Action Port : ActionPort  ActionType=else
  " Wrapping" : Subsystem
  Add1 : Sum  RequirementInfo="{'linktype_rmi_doors' '0000bb46 (/E-STEER Core/SubSystem Specifications/Application Functions/SF99/SF107A Cogging and Ripple Command Generation)' '#SF107A_50' 'true' 'REQ:  SF107A_50' '' } %GIDa_f02d4a4d_036f_4693_b593_d5ebaac87e78"
  Add8 : Sum  RequirementInfo="{'linktype_rmi_doors' '0000bb46 (/E-STEER Core/SubSystem Specifications/Application Functions/SF99/SF107A Cogging and Ripple Command Generation)' '#SF107A_50' 'true' 'REQ:  SF107A_50' '' } %GIDa_eedba08f_ca99_41b1_8c3b_095858d88b6c"
  CoggTq Computation : Subsystem
  Constant2 : Constant  Value=ONEOVER2PI_ULS_F32
  CopyRight2 : Subsystem  Description=|  mask(Copyright Information){none=on}
      | Copyright info block.                                               
      |                                                                     
      | Place copyright information at the top of every subsystem in design.
      mask prompts: none "No parameters"
      mask help: Place copyright information at the top of every subsystem in design.
      mask Display:
      | NxtrConf = 'Nexteer Confidential';
      | 
      | sys = bdroot; %handle for the current model ("system")
      | first = get_param(sys,'Created');
      | if(isempty(first))
      |     first = datestr(now,'yyyy');
      | else
      |     first = first(end-3:end);  %year is last four digits
      | end
      | 
      | last = get_param(sys,'LastModifiedDate');
      | if isempty(last)
      |     last = datestr(now,'yyyy');
      | else
      |     last = last(end-3:end);
      | end
      | 
      | if strcmp(first,last)
      |     fprintf('%s -- Copyright %s Nexteer',NxtrConf,first)
      | else
      |     fprintf('%s -- %s%s- %s Nexteer',NxtrConf,char(169),first,last)
      | end
  FloatToFixd_u16_f32 : FloatToFixd/FloatToFixd_u16_f32  Param1=16
  MotElecMeclPolarity Compensating : Subsystem
  Product : Product
  TqRpl Computation : Subsystem
  MotCurrQaxRplCmd : Outport
  MotCurrQaxCoggCmd : Outport  Port=2
  wires:
  Add8/1 -> " Wrapping"/1(MotAgElecDly)
  MotElecMeclPolarity Compensating/1(MotElecMeclPolarityCmp) -> Add8/2
  MotCurrQaxMotTqGain/1 -> [MotCurrQaxMotTqGain]
  MotCtrlMotAgElecDly/1 -> Product/1
  MotCtrlMotElecMeclPolarity/1 -> MotElecMeclPolarity Compensating/1(MotElecMeclPolarity)
  MotTqRplCoggOrder1Pha/1 -> TqRpl Computation/3(MotTqRplCoggOrder1Pha)
  MotTqRplCoggOrder2Pha/1 -> TqRpl Computation/4(MotTqRplCoggOrder2Pha)
  MotTqRplCoggOrder3Pha/1 -> TqRpl Computation/5(MotTqRplCoggOrder3Pha)
  MotTqRplCoggOrder1Mgn/1 -> TqRpl Computation/6(MotTqRplCoggOrder1Mgn)
  MotTqRplCoggOrder2Mgn/1 -> TqRpl Computation/7(MotTqRplCoggOrder2Mgn)
  MotTqRplCoggOrder3Mgn/1 -> TqRpl Computation/8(MotTqRplCoggOrder3Mgn)
  [CorrdElecPosn] -> TqRpl Computation/1(CorrdElecPosn)
  TqRpl Computation/1(MotCtrlMotCurrQaxRplCmd) -> MotCurrQaxRplCmd/1
  [MotCurrQaxMotTqGain] -> TqRpl Computation/2(CurrQaxMotTqGain)
  CoggTq Computation/1(MotCurrQaxCoggCmd) -> MotCurrQaxCoggCmd/1
  [MotCurrQaxMotTqGain] -> CoggTq Computation/2(MotCurrQaxMotTqGain)
  [CorrdElecPosn] -> CoggTq Computation/1(CorrdElecPosn)
  FloatToFixd_u16_f32/1 -> Add1/1
  Add1/1 -> [CorrdElecPosn]
  MotCtrlMotAgElec/1 -> Add1/2
  Constant2/1 -> Product/2
  Product/1 -> Add8/1
  " Wrapping"/1(MotAgElecDlyCalcd) -> FloatToFixd_u16_f32/1

== system SF107A_MotRplCoggCmd/MotRplCoggCmd/MotRplCoggCmdPer1/Set to 0 ==
  Action Port : ActionPort  ActionType=then
  Constant : Constant  Value=0  OutDataTypeStr=single
      settings: AttributesFormatString=%<OutDataTypeStr>
  Constant1 : Constant  Value=0  OutDataTypeStr=single
      settings: AttributesFormatString=%<OutDataTypeStr>
  CopyRight2 : Subsystem  Description=|  mask(Copyright Information){none=on}
      | Copyright info block.                                               
      |                                                                     
      | Place copyright information at the top of every subsystem in design.
      mask prompts: none "No parameters"
      mask help: Place copyright information at the top of every subsystem in design.
      mask Display:
      | NxtrConf = 'Nexteer Confidential';
      | 
      | sys = bdroot; %handle for the current model ("system")
      | first = get_param(sys,'Created');
      | if(isempty(first))
      |     first = datestr(now,'yyyy');
      | else
      |     first = first(end-3:end);  %year is last four digits
      | end
      | 
      | last = get_param(sys,'LastModifiedDate');
      | if isempty(last)
      |     last = datestr(now,'yyyy');
      | else
      |     last = last(end-3:end);
      | end
      | 
      | if strcmp(first,last)
      |     fprintf('%s -- Copyright %s Nexteer',NxtrConf,first)
      | else
      |     fprintf('%s -- %s%s- %s Nexteer',NxtrConf,char(169),first,last)
      | end
  MotCurrQaxRplCmd : Outport
  MotCurrQaxCoggCmd : Outport  Port=2
  wires:
  Constant/1 -> MotCurrQaxRplCmd/1
  Constant1/1 -> MotCurrQaxCoggCmd/1

== system SF107A_MotRplCoggCmd/MotRplCoggCmd/SetMotCoggCmdPrm/CopyRight1 ==

== system SF107A_MotRplCoggCmd/MotRplCoggCmd/SetMotCoggCmdPrm/For Iterator Subsystem1 ==
  MotCoggCmdY : Inport
  Idx : Inport  Port=2
  ItrnIdxCon : Inport  Port=3
  Add : Sum
  Assignment : Assignment  IndexMode=Zero-based  IndexOptions=Index vector (port)  Indices=1  OutputSizes=128
  CopyRight1 : Subsystem  Description=|  mask(Copyright Information){none=on}
      | Copyright info block.                                               
      |                                                                     
      | Place copyright information at the top of every subsystem in design.
      mask prompts: none "No parameters"
      mask help: Place copyright information at the top of every subsystem in design.
      mask Display:
      | NxtrConf = 'Nexteer Confidential';
      | 
      | sys = bdroot; %handle for the current model ("system")
      | first = get_param(sys,'Created');
      | if(isempty(first))
      |     first = datestr(now,'yyyy');
      | else
      |     first = first(end-3:end);  %year is last four digits
      | end
      | 
      | last = get_param(sys,'LastModifiedDate');
      | if isempty(last)
      |     last = datestr(now,'yyyy');
      | else
      |     last = last(end-3:end);
      | end
      | 
      | if strcmp(first,last)
      |     fprintf('%s -- Copyright %s Nexteer',NxtrConf,first)
      | else
      |     fprintf('%s -- %s%s- %s Nexteer',NxtrConf,char(169),first,last)
      | end
  Data Store Read2 : DataStoreRead  DataStoreName=MotCoggCmdY
  Data Store Write : DataStoreWrite  DataStoreName=MotCoggCmdY
  For Iterator : ForIterator  IterationSource=external  IterationLimit=127  IndexMode=Zero-based  IterationVariableDataType=int16
  Product : Product  OutDataTypeStr=int16
  Selector : Selector  IndexMode=Zero-based  InputPortWidth=128  IndexOptions=Index vector (port)  Indices=[1 3]  OutputSizes=1
  wires:
  Data Store Read2/1 -> Assignment/1
  Product/1 -> Add/2
  MotCoggCmdY/1 -> Selector/1
  Assignment/1 -> Data Store Write/1
  For Iterator/1 -> Add/1, Selector/2
  Idx/1 -> Product/2
  ItrnIdxCon/1 -> Product/1, For Iterator/1
  Add/1 -> Assignment/3
  Selector/1 -> Assignment/2

== system SF107A_MotRplCoggCmd/MotRplCoggCmd/GetMotCoggCmdPrm/For Iterator Subsystem/CopyRight1 ==

== system SF107A_MotRplCoggCmd/MotRplCoggCmd/MotRplCoggCmdInit1/NVM is NOT okay/CopyRight2 ==

== system SF107A_MotRplCoggCmd/MotRplCoggCmd/MotRplCoggCmdInit1/NVM is NOT okay/For Iterator Subsystem ==
  In1 : Inport
  Assignment : Assignment  IndexMode=Zero-based  OutputInitialize=Specify size for each dimension in table  IndexOptions=Index vector (port)  Indices=1  OutputSizes=512
  Constant : Constant  OutDataTypeStr=single
  CopyRight2 : Subsystem  Description=|  mask(Copyright Information){none=on}
      | Copyright info block.                                               
      |                                                                     
      | Place copyright information at the top of every subsystem in design.
      mask prompts: none "No parameters"
      mask help: Place copyright information at the top of every subsystem in design.
      mask Display:
      | NxtrConf = 'Nexteer Confidential';
      | 
      | sys = bdroot; %handle for the current model ("system")
      | first = get_param(sys,'Created');
      | if(isempty(first))
      |     first = datestr(now,'yyyy');
      | else
      |     first = first(end-3:end);  %year is last four digits
      | end
      | 
      | last = get_param(sys,'LastModifiedDate');
      | if isempty(last)
      |     last = datestr(now,'yyyy');
      | else
      |     last = last(end-3:end);
      | end
      | 
      | if strcmp(first,last)
      |     fprintf('%s -- Copyright %s Nexteer',NxtrConf,first)
      | else
      |     fprintf('%s -- %s%s- %s Nexteer',NxtrConf,char(169),first,last)
      | end
  Data Store Write1 : DataStoreWrite  DataStoreName=MotCoggCmdY
  FloatToFixd_s16_f32 : FloatToFixd/FloatToFixd_s16_f32  Param1=14
  For Iterator : ForIterator  IterationSource=external  IterationLimit=512  IndexMode=Zero-based  IterationVariableDataType=int16
  wires:
  In1/1 -> For Iterator/1
  For Iterator/1 -> Assignment/2
  Assignment/1 -> Data Store Write1/1
  FloatToFixd_s16_f32/1 -> Assignment/1
  Constant/1 -> FloatToFixd_s16_f32/1

== system SF107A_MotRplCoggCmd/MotRplCoggCmd/MotRplCoggCmdPer1/Regular Calculation/ Wrapping ==
  note: Output 0
  note: Output 1 MotRev
  MotAgElecDly : Inport
  Add2 : Sum  RequirementInfo="{'linktype_rmi_doors' '0000bb46 (/E-STEER Core/SubSystem Specifications/Application Functions/SF99/SF107A Cogging and Ripple Command Generation)' '#SF107A_51' 'true' 'REQ:  SF107A_51' '' } %GIDa_ff3c4045_8256_4ebe_a8d4_67c81565112e"
  Constant1 : Constant  Value=0  OutDataTypeStr=single
      settings: AttributesFormatString=%<OutDataTypeStr>
  CopyRight2 : Subsystem  Description=|  mask(Copyright Information){none=on}
      | Copyright info block.                                               
      |                                                                     
      | Place copyright information at the top of every subsystem in design.
      mask prompts: none "No parameters"
      mask help: Place copyright information at the top of every subsystem in design.
      mask Display:
      | NxtrConf = 'Nexteer Confidential';
      | 
      | sys = bdroot; %handle for the current model ("system")
      | first = get_param(sys,'Created');
      | if(isempty(first))
      |     first = datestr(now,'yyyy');
      | else
      |     first = first(end-3:end);  %year is last four digits
      | end
      | 
      | last = get_param(sys,'LastModifiedDate');
      | if isempty(last)
      |     last = datestr(now,'yyyy');
      | else
      |     last = last(end-3:end);
      | end
      | 
      | if strcmp(first,last)
      |     fprintf('%s -- Copyright %s Nexteer',NxtrConf,first)
      | else
      |     fprintf('%s -- %s%s- %s Nexteer',NxtrConf,char(169),first,last)
      | end
  If Action Subsystem1 : Subsystem  RequirementInfo="{'linktype_rmi_doors' '0000bb46 (/E-STEER Core/SubSystem Specifications/Application Functions/SF99/SF107A Cogging and Ripple Command Generation)' '#SF107A_51' 'true' 'REQ:  SF107A_51' '' } %GIDa_9a8cd899_f791_44cf_843a_37fc84c7b667"  TreatAsAtomicUnit=on
  If Action Subsystem5 : Subsystem  RequirementInfo="{'linktype_rmi_doors' '0000bb46 (/E-STEER Core/SubSystem Specifications/Application Functions/SF99/SF107A Cogging and Ripple Command Generation)' '#SF107A_51' 'true' 'REQ:  SF107A_51' '' } %GIDa_d1e18887_de06_47f6_b182_a182110d3317"  TreatAsAtomicUnit=on
  If1 : If  RequirementInfo="{'linktype_rmi_doors' '0000bb46 (/E-STEER Core/SubSystem Specifications/Application Functions/SF99/SF107A Cogging and Ripple Command Generation)' '#SF107A_51' 'true' 'REQ:  SF107A_51' '' } %GIDa_3558578c_ba96_49f5_bf07_e1bba3bbd8da"  IfExpression=u1
  Merge2 : Merge  RequirementInfo="{'linktype_rmi_doors' '0000bb46 (/E-STEER Core/SubSystem Specifications/Application Functions/SF99/SF107A Cogging and Ripple Command Generation)' '#SF107A_51' 'true' 'REQ:  SF107A_51' '' } %GIDa_fc51fd5d_24c6_40ae_984e_dc989b6957ae"
  Relational Operator : RelationalOperator  RequirementInfo="{'linktype_rmi_doors' '0000bb46 (/E-STEER Core/SubSystem Specifications/Application Functions/SF99/SF107A Cogging and Ripple Command Generation)' '#SF107A_51' 'true' 'REQ:  SF107A_51' '' } %GIDa_e844345b_eb40_4069_a20e_5c6eb8b33120"  Operator=<  OutDataTypeStr=boolean
  MotAgElecDlyCalcd : Outport
  wires:
  If1/2 -> If Action Subsystem5/Action
  If Action Subsystem1/1(Out1) -> Merge2/1
  If Action Subsystem5/1(Out1) -> Merge2/2
  Relational Operator/1 -> If1/1
  Constant1/1 -> Relational Operator/2
  Merge2/1 -> Add2/1
  If1/1 -> If Action Subsystem1/Action
  MotAgElecDly/1 -> Add2/2, Relational Operator/1
  Add2/1 -> MotAgElecDlyCalcd/1
